simulink model "CH6_1"  (Simulink 5.0)
settings: Solver=ode23tb  SolverMode=SingleTasking  StartTime=0.0  StopTime=0.03  RelTol=1e-5
libraries: powerlib2 x16
Description:
  | 高苑科技大學 電機系
  | 電力電子實驗室
settings Model: Creator=徐瑞隆老師  LastModifiedBy=ELECTRONIC  ExtModeTrigMode=oneshot  ExtModeArmWhenConnect=off  LimitDataPoints=off  BooleanDataType=off  RTWTemplateMakefile=grt_unix.tmf

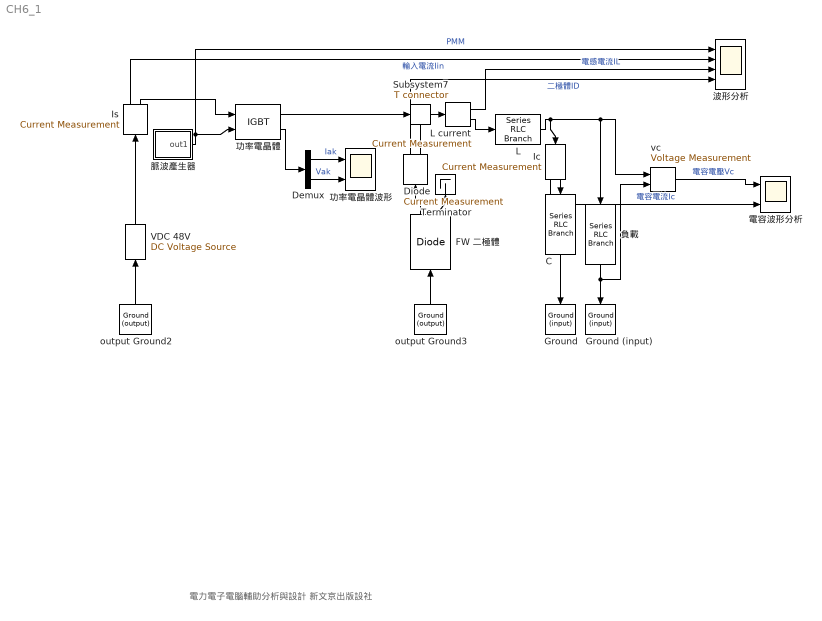
== system CH6_1 ==
  note: 電力電子電腦輔助分析與設計 新文京出版設社
  " 負載   " : powerlib2/Elements/Series RLC Branch  Tag=PoWeRsYsTeMbLoCk  Orientation=down  a=20  b=0  c=inf  mesure=None  PSBOutputType=1
  C : powerlib2/Elements/Series RLC Branch  Tag=PoWeRsYsTeMbLoCk  Orientation=down  a=0  b=0  c=100e-6  mesure=None  PSBOutputType=1
  Demux : Demux  Outputs=2
  Diode : powerlib2/Measurements/Current Measurement  Tag=PoWeRsYsTeMmEaSuReMeNt  Orientation=up  PhasorSimulation=off  OutputType=Magnitude  PSBOutputType=01  PSBequivalent=0
  FW 二極體 : powerlib2/Power Electronics/Diode  Tag=PoWeRsYsTeMbLoCk  Orientation=up  Ron=0.01  Lon=1e-6  Vf=0  IC=0  Rs=1000  Cs=0.1e-6  PSBOutputType=10
  Ground : powerlib2/Connectors/Ground (input)  Tag=PoWeRsYsTeMbLoCk  Orientation=down
  Ground (input) : powerlib2/Connectors/Ground (input)  Tag=PoWeRsYsTeMbLoCk  Orientation=down
  Ic : powerlib2/Measurements/Current Measurement  Tag=PoWeRsYsTeMmEaSuReMeNt  Orientation=down  PhasorSimulation=off  OutputType=Magnitude  PSBOutputType=01  PSBequivalent=0
  Is : powerlib2/Measurements/Current Measurement  Tag=PoWeRsYsTeMmEaSuReMeNt  Orientation=up  PhasorSimulation=off  OutputType=Magnitude  PSBOutputType=01  PSBequivalent=0
  L : powerlib2/Elements/Series RLC Branch  Tag=PoWeRsYsTeMbLoCk  a=0  b=400e-6  c=inf  mesure=None  PSBOutputType=1
  L current : powerlib2/Measurements/Current Measurement  Tag=PoWeRsYsTeMmEaSuReMeNt  PhasorSimulation=off  OutputType=Magnitude  PSBOutputType=01  PSBequivalent=0
  Subsystem7 : powerlib2/Connectors/T connector  Tag=PoWeRsYsTeMbLoCk  PSBOutputType=1
  Terminator : Terminator
      settings: Orientation=up
  VDC 48V : powerlib2/Electrical Sources/DC Voltage Source  Tag=PoWeRsYsTeMbLoCk  Orientation=up  V=48  mesure=None  PSBOutputType=1
  output Ground2 : powerlib2/Connectors/Ground (output)  Tag=PoWeRsYsTeMbLoCk  Orientation=up  PSBOutputType=1
  output Ground3 : powerlib2/Connectors/Ground (output)  Tag=PoWeRsYsTeMbLoCk  Orientation=up  PSBOutputType=1
  vc : powerlib2/Measurements/Voltage Measurement  Tag=PoWeRsYsTeMmEaSuReMeNt  PhasorSimulation=off  OutputType=Magnitude  PSBOutputType=0  PSBequivalent=0
  功率電晶體 : powerlib2/Power Electronics/IGBT  Tag=PoWeRsYsTeMbLoCk  Ron=0.001  Lon=1e-6  Vf=0  Tf=1e-6  Tt=2e-6  IC=0  Rs=inf  Cs=0  PSBOutputType=10
  功率電晶體波形 : Scope  NumInputPorts=2
      settings: TimeRange=0.01  YMin=0~0  YMax=60~300  DataFormat=Array  MaxDataPoints=500000
  波形分析 : Scope  NumInputPorts=4
      settings: TimeRange=0.01  YMin=-50~-100~-5~-5  YMax=50~200~5~5  DataFormat=Array  MaxDataPoints=1500
  脈波產生器 : Subsystem  mask(Pulse Generator){period=1/20000, duty=40, amplitude=1, start=0}
      mask prompts: period "Period (secs):"; duty "Duty cycle (% of period):"; start "Start time:"
      mask help: Pulse Generator
      mask Help: Pulse generator which ensures pulse transitions are hit. Provides a vector of pulses when the height is entered as a vector.  Unmask to see how it works.
      mask Display: plot(0,0,100,100,[95,90,90,75,75,60,60,45,45,30,30,15,15,5],[25,25,75,75,25,25,75,75,25,25,75,75,25,25]);
  電容波形分析 : Scope  NumInputPorts=2
      settings: TimeRange=0.01  YMin=-50~-100  YMax=50~200  DataFormat=Array
  wires:
  output Ground3/1 -> FW 二極體/1
  C/1 -> Ground/1
  output Ground2/1 -> VDC 48V/1
  Subsystem7/1 -> L current/1
  脈波產生器/1(out1) -> 功率電晶體/2, 波形分析/1  "PMM"
  功率電晶體/1 -> Subsystem7/1
  FW 二極體/2 -> Terminator/1
  Demux/1 -> 功率電晶體波形/1  "Iak"
  Demux/2 -> 功率電晶體波形/2  "Vak"
  L current/2 -> L/1
  L/1 -> " 負載   "/1, vc/1, Ic/1
  " 負載   "/1 -> Ground (input)/1, vc/2
  功率電晶體/2 -> Demux/1
  Diode/2 -> Subsystem7/Enable
  FW 二極體/1 -> Diode/1
  Ic/2 -> C/1
  VDC 48V/1 -> Is/1
  Is/2 -> 功率電晶體/1
  Is/1 -> 波形分析/2  "輸入電流Iin"
  Diode/1 -> 波形分析/4  "二極體ID"
  L current/1 -> 波形分析/3  "電感電流IL"
  vc/1 -> 電容波形分析/1  "電容電壓Vc"
  Ic/1 -> 電容波形分析/2  "電容電流Ic"

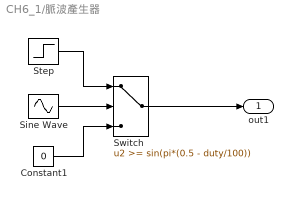
== system CH6_1/脈波產生器 ==
  Constant1 : Constant  Value=0
  Sine Wave : Sin  Frequency=2*pi./period  Phase=-2*pi*(start./period + duty/200 - 1/4)  SampleTime=0
  Step : Step  Time=start  After=amplitude  SampleTime=0
  Switch : Switch  Threshold=sin(pi*(0.5 - duty/100))  SaturateOnIntegerOverflow=on  InputSameDT=on
  out1 : Outport  InitialOutput=0
  wires:
  Step/1 -> Switch/1
  Constant1/1 -> Switch/3
  Switch/1 -> out1/1
  Sine Wave/1 -> Switch/2
